simulink model "simplified_sim_20181"  (R2018b)
settings: Solver=VariableStepAuto  StartTime=0.0  StopTime=10.0  RelTol=1e-3
libraries: MEKF_conversion_lib x1, Environment_lib x1, MEKF_lib x1, Sensors_Lib x1, satelliteDynamics_lib x1
settings Model: Creator=satcave1  LastModifiedBy=satcave1

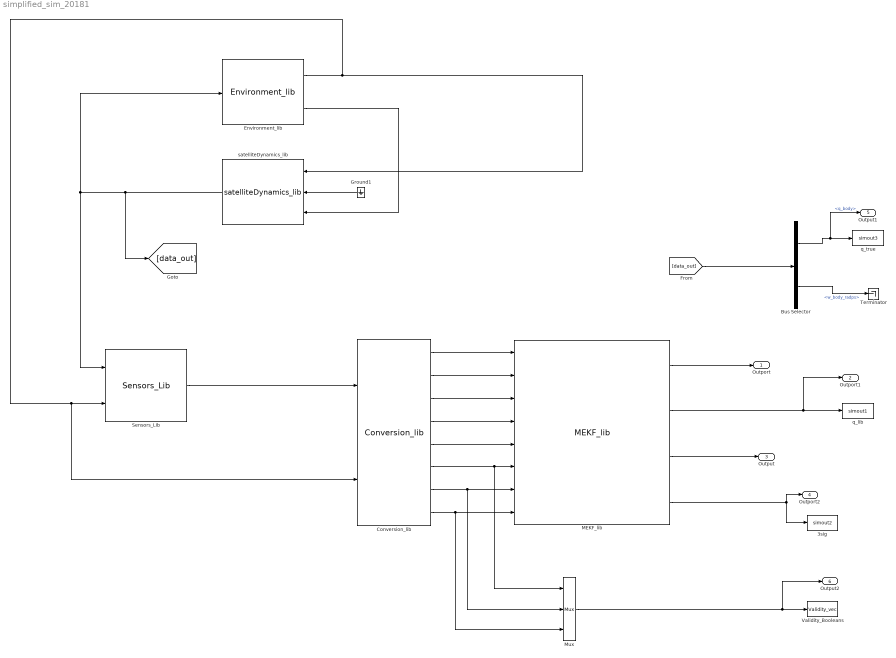
== system simplified_sim_20181 ==
  3sig : ToWorkspace  VariableName=simout2  SaveFormat=Timeseries  SampleTime=-1
  Bus Selector : BusSelector  OutputSignals=q_body,w_body_radps
  Conversion_lib : MEKF_conversion_lib/Conversion_lib  SystemSampleTime=-1
  Environment_lib : Environment_lib/Environment_lib  SystemSampleTime=-1
  Ground1 : Ground
  MEKF_lib : MEKF_lib/MEKF_lib  SystemSampleTime=-1
  Mux : Mux  Inputs=3
  Sensors_Lib : Sensors_Lib/Sensors_Lib  SystemSampleTime=-1
  Terminator : Terminator
  Validity_Booleans : ToWorkspace  VariableName=Validity_vec  SaveFormat=Timeseries  SampleTime=-1
  q_lib : ToWorkspace  VariableName=simout1  SaveFormat=Timeseries  SampleTime=-1
  q_true : ToWorkspace  VariableName=simout3  SaveFormat=Timeseries  SampleTime=-1
  satelliteDynamics_lib : satelliteDynamics_lib/satelliteDynamics_lib  SystemSampleTime=-1
  Outport : Outport
  Outport1 : Outport  Port=2
  Output : Outport  Port=3
  Outport2 : Outport  Port=4
  Output1 : Outport  Port=5
  Output2 : Outport  Port=6
  wires:
  satelliteDynamics_lib/1 -> [data_out], Environment_lib/1, Sensors_Lib/1
  Ground1/1 -> satelliteDynamics_lib/2
  Environment_lib/2 -> satelliteDynamics_lib/3
  MEKF_lib/2 -> Outport1/1, q_lib/1
  MEKF_lib/1 -> Outport/1
  MEKF_lib/4 -> 3sig/1, Outport2/1
  MEKF_lib/3 -> Output/1
  [data_out] -> Bus Selector/1
  Bus Selector/1 -> Output1/1, q_true/1  "<q_body>"
  Bus Selector/2 -> Terminator/1  "<w_body_radps>"
  Environment_lib/1 -> Conversion_lib/2, Sensors_Lib/2, satelliteDynamics_lib/1
  Conversion_lib/1 -> MEKF_lib/1
  Conversion_lib/2 -> MEKF_lib/2
  Conversion_lib/3 -> MEKF_lib/3
  Conversion_lib/4 -> MEKF_lib/4
  Conversion_lib/5 -> MEKF_lib/5
  Conversion_lib/6 -> Mux/1, MEKF_lib/6
  Conversion_lib/7 -> Mux/2, MEKF_lib/7
  Conversion_lib/8 -> Mux/3, MEKF_lib/8
  Sensors_Lib/1 -> Conversion_lib/1
  Mux/1 -> Output2/1, Validity_Booleans/1
